simulink model "model2bf_Chikri"  (R2024b)
settings: Solver=ode4  StartTime=0.0  StopTime=20  FixedStep=2e-3  MaxStep=1e-1  RelTol=1e-3
values from neighbouring files (symbols this model uses):
  Aero = struct    [model2_dim.m]    (also in model2_dim_Chikri.m)
  brake = struct    [model2_dim.m]    (also in model2_dim_Chikri.m)
  drivetrain = struct    [model2_dim.m]    (also in model2_dim_Chikri.m)
  g = 9.81    [model2_dim.m]    (also in model2_dim_Chikri.m)
  G29 = struct    [model2_dim.m]    (also in model2_dim_Chikri.m)
  hub_offset = 2.5    [model2_dim.m]    (also in model2_dim_Chikri.m)
  motor = struct    [model2_dim.m]    (also in model2_dim_Chikri.m)
  slope_angle = 0    [model2_dim.m]    (also in model2_dim_Chikri.m)
  suspension = struct    [model2_dim.m]    (also in model2_dim_Chikri.m)
  tyre = struct    [model2_dim.m]    (also in model2_dim_Chikri.m)
  vehicle = struct    [Dimesnsion.m]    (also in model2_dim.m; model2_dim_Chikri.m)
undefined symbols (not defined in the file or in its folder): table, wheel, X, Y, Z
libraries: sm_lib x154, nesl_utility x46, simulink x8, slrealtimeG29lib x1, Contact_Forces_Lib x1
(part 1 of 6)
settings Model: Creator=francescovalentia  LastModifiedBy=chikr
settings SolverCC: ConcurrentTasks=on  SolverResetMethod=Robust  PositivePriorityOrder=on
settings DebuggingCC: ReadBeforeWriteMsg=DisableAll  WriteAfterWriteMsg=DisableAll  WriteAfterReadMsg=DisableAll  TasksWithSamePriorityMsg=none
settings HardwareCC: ProdBitPerLong=64  ProdLongLongMode=on  ProdHWDeviceType=Intel->x86-64 (Linux 64)
settings ModelReferenceCC: UpdateModelReferenceTargets=IfOutOfDate
settings SFSimCC: SFSimEcho=off
settings RTWCC: Description=Speedgoat Real-Time Target Machine  SystemTargetFile=speedgoat.tlc  TemplateMakefile=slrealtime_default_tmf  Toolchain=Simulink Real-Time Toolchain  BuildConfiguration=Faster Runs  CodeExecutionProfiling=on  TargetLang=C++
settings SimulinkRealTimeTargetCC: InstructionSetFMA=off  LogToMDFFile=off  SLRTForcePollingMode=on  UseGCCFastMath=on

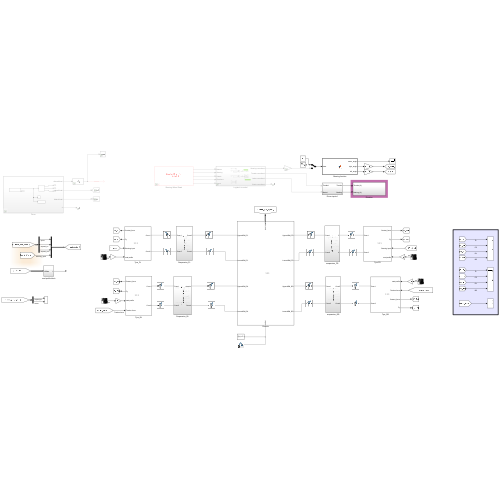
[thumbnail: Simulink's stored preview of the top-level diagram]
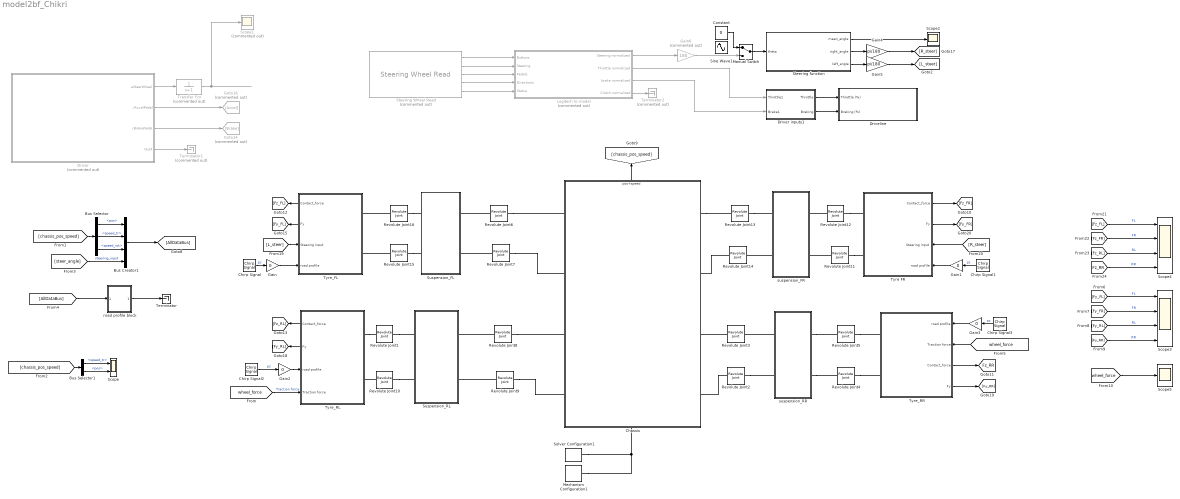
== system model2bf_Chikri ==
  Bus Creator1 : BusCreator  Inputs=4
  Bus Selector : BusSelector  OutputSignals=pos,speed_tr,speed_rot
  Bus Selector1 : BusSelector  OutputSignals=speed_tr,pos
  Chassis : Subsystem
      settings: PortSchema="{\"entries\":[{\"content\":{\"sides\":[{\"content\":{\"connectorIds\":[\"LConn1\",\"LConn2\",\"LConn3\",\"LConn4\"]},\"type\":\"ConnectorPlacement.EquallySpacedRectSide\",\"uuid\":\"90a4177c-ee01-4ca1-ac59-ac8cd2430efa\"},{\"content\":{\"connectorIds\":[\"RConn1\",\"RConn2\",\"RConn3\",\"RConn4\"],\"side\":\"RIGHT\"},\"type\":\"ConnectorPlacement.EquallySpacedRectSide\",\"uuid\":\"edda8be8-83bb-4564-b638-4691278f5470\"},{\"content\":{\"connectorIds\":[\"Out1\"],\"side\":\"TOP\"},\"type\":\"ConnectorPlacement.EquallySpacedRectSide\",\"uuid\":\"1072aa4a-3e89-42c9-923f-70cc607d97c1\"},{\"content\":{\"connectorIds\":[\"RConn5\"],\"side\":\"BOTTOM\"},\"type\":\"ConnectorPlacement.EquallySpacedRectSide\",\"uuid\":\"b3a5ffc1-0a8d-40b3-87bf-50b9fb640548\"}]},\"type\":\"ConnectorPlacement.EquallySpacedConnector\",\"uuid\":\"42fa0a11-996d-4d38-ac5b-1505bea5ca1e\"}],\"packageUris\":[\"http://schema.mathworks.com/mf0/Connector/R2020b\"],\"version\":\"1.0\"}"
      mask Display: image('Screenshot 2025-03-01 at 00.26 Background Removed.44.png');
  Chirp Signal{,1..3} (4 alike) : simulink/Sources/Chirp Signal  f1=0.01  T=10  f2=10
  Constant : Constant  Value=0
  Driveline : Subsystem
  Driver : Subsystem  Commented=on
  Driver inputs1 : Subsystem
  Gain{,1..3} (4 alike) : Gain  Gain=0
  Gain4 : Gain  Gain=pi/180
  Gain5 : Gain  Gain=pi/180
  Gain6 : Gain  Commented=on  Gain=180
  Goto14 : Goto  Commented=on  GotoTag=Brake
  Goto16 : Goto  Commented=on  GotoTag=Accel
  Logitech to model : Subsystem  Commented=on
  Manual Switch : ManualSwitch
  Mechanism Configuration1 : sm_lib/Utilities/Mechanism Configuration  UniformGravity=Constant  GravityVector=[0 0 -9.80665]  GravityVectorUnits=m/s^2  LinearizationDelta=0.001  JointModeTransitionNonlinearIterations=2
  Revolute Joint{1..16} (16 alike) : sm_lib/Joints/Revolute Joint  JointMode=Normal  CompositeWrenchDir=FollowerOnBase  CompositeWrenchFrame=BaseFrame  SenseConstraintForce=off  SenseConstraintTorque=off  SenseTotalForce=off  SenseTotalTorque=off  PositionTargetSpecify=off  PositionTargetPriority=High  PositionTargetValue=0  PositionTargetValueUnits=deg  VelocityTargetSpecify=off  VelocityTargetPriority=High  VelocityTargetValue=0  VelocityTargetValueUnits=deg/s  EquilibriumPosition=0  EquilibriumPositionUnits=deg  SpringStiffness=0  SpringStiffnessUnits=N*m/deg  DampingCoefficient=0  DampingCoefficientUnits=N*m/(deg/s)  LowerLimitSpecify=off  LowerLimitBound=-90  LowerLimitBoundUnits=deg  LowerLimitStiffness=1e4  LowerLimitStiffnessUnits=N*m/deg  LowerLimitDamping=10  LowerLimitDampingUnits=N*m/(deg/s)  LowerLimitTransitionRegionWidth=0.1  LowerLimitTransitionRegionWidthUnits=deg  UpperLimitSpecify=off  UpperLimitBound=90  UpperLimitBoundUnits=deg  UpperLimitStiffness=1e4  UpperLimitStiffnessUnits=N*m/deg  UpperLimitDamping=10  UpperLimitDampingUnits=N*m/(deg/s)  UpperLimitTransitionRegionWidth=0.1  UpperLimitTransitionRegionWidthUnits=deg  TorqueActuationMode=NoTorque  MotionActuationMode=ComputedMotion  SensePosition=off  SenseVelocity=off  SenseAcceleration=off  SenseTorqueForce=off  SenseLowerLimitTorqueForce=off  SenseUpperLimitTorqueForce=off
  Scope : Scope  NumInputPorts=2
  Scope1 : Scope  Commented=on
  Scope2 : Scope
  Scope3 : Scope  NumInputPorts=4
  Scope4 : Scope  NumInputPorts=4
  Scope5 : Scope
  Sine Wave1 : Sin  Amplitude=30  Frequency=1*2*pi  SampleTime=0
  Solver Configuration1 : nesl_utility/Solver Configuration  PhysicalDomain=network_engine_domain  SubClassName=solver  LeftPortType=input  RightPortType=generic  Tones=[]  Harmonics=[]  SimulateNoise=off  Profile=off  UseLocalSampling=off  EnableSwitchedLinearOptims=on  FrequencyDomain=off  UseCCode=off  RelTol=0.001  AbsTol=0.001  MinStep=1e-09  ToWorkspace=off  RevertToSquareIcSolve=off  NumHomotopyIterations=100  PhasorMode=off  PhasorModeNumHarmonics=1  ConsistencySolver=NEWTON_XTOL_AFTER_FTOL  IndexReductionMethod=DerivativeReplacement  DoDC=off  ResidualTolerance=1e-09  ConsistencyTolSource=GLOBAL  ConsistencyAbsTol=0.001  ConsistencyRelTol=0.001  ConsistencyTolFactor=0.02  UseLocalSolver=off  LocalSolverChoice=NE_BACKWARD_EULER_ADVANCER  ResolveIndetEquations=on  FunctionEvalNumThread=1  LocalSolverSampleTime=0.001  DoFixedCost=off  MaxNonlinIter=3  MaxModeIter=2  ComputeImpulses=off  ImpulseIterations=2  LinearAlgebra=auto  LinearAlgebraNumThread=0  EquationFormulation=NE_TIME_EF  DelaysMemoryBudget=1024  AutomaticFiltering=on  FilteringTimeConstant=0.001  PartitionStorageMethod=AS_NEEDED  PartitionMemoryBudget=1024  PartitionMethod=ROBUST  MultibodyUseLocalSolver=off  MultibodyLocalSolverChoice=ODE1  MultibodyLocalSolverSampleTime=0.001
  Steering Wheel Read : slrealtimeG29lib/Steering Wheel Read  Commented=on  sampleTime=-1
  Steering function : MATLAB Function  TreatAsAtomicUnit=on
  Suspension_FL : Subsystem
  Suspension_RL : Subsystem
  Terminator : Terminator
  Terminator1 : Terminator  Commented=on
  Terminator2 : Terminator  Commented=on
  Transfer Fcn : TransferFcn  Commented=on  Denominator=[1 1]
  Tyre FR : Subsystem
      settings: PortSchema="{\"entries\":[{\"content\":{\"sides\":[{\"content\":{\"connectorIds\":[\"LConn1\",\"LConn2\"]},\"type\":\"ConnectorPlacement.EquallySpacedRectSide\",\"uuid\":\"7590dd46-fd1e-41dd-87a1-62791c0994cf\"},{\"content\":{\"connectorIds\":[\"Out1\",\"Out2\",\"In1\",\"In2\"],\"side\":\"RIGHT\"},\"type\":\"ConnectorPlacement.EquallySpacedRectSide\",\"uuid\":\"4353fa18-87e5-46ea-8b75-e97175ca5d0d\"},{\"content\":{\"side\":\"TOP\"},\"type\":\"ConnectorPlacement.EquallySpacedRectSide\",\"uuid\":\"fb2fe8ac-4791-48d4-8005-7292892240b2\"}]},\"type\":\"ConnectorPlacement.EquallySpacedConnector\",\"uuid\":\"4af72fb6-bebe-4fb7-b2ff-d8311ffebfc8\"}],\"packageUris\":[\"http://schema.mathworks.com/mf0/Connector/R2020b\"],\"version\":\"1.0\"}"
      mask Display: image('tire.jpg');
  Tyre_FL : Subsystem
      settings: PortSchema="{\"entries\":[{\"content\":{\"sides\":[{\"content\":{\"connectorIds\":[\"Out1\",\"Out2\",\"In1\",\"In2\"]},\"type\":\"ConnectorPlacement.EquallySpacedRectSide\",\"uuid\":\"bd1bd92e-18de-4596-8220-631603715178\"},{\"content\":{\"connectorIds\":[\"RConn1\",\"RConn2\"],\"side\":\"RIGHT\"},\"type\":\"ConnectorPlacement.EquallySpacedRectSide\",\"uuid\":\"e020c9fe-d1b2-4d80-947d-230813d0e146\"},{\"content\":{\"side\":\"TOP\"},\"type\":\"ConnectorPlacement.EquallySpacedRectSide\",\"uuid\":\"ef1b0779-8900-451f-8b58-5aab45ce88d5\"}]},\"type\":\"ConnectorPlacement.EquallySpacedConnector\",\"uuid\":\"d082f1b5-3bbc-432b-b3b6-f4f290eb68cb\"}],\"packageUris\":[\"http://schema.mathworks.com/mf0/Connector/R2020b\"],\"version\":\"1.0\"}"
      mask Display: image('tire.jpg');
  Tyre_RL : Subsystem
      settings: PortSchema="{\"entries\":[{\"content\":{\"sides\":[{\"content\":{\"connectorIds\":[\"Out1\",\"Out2\",\"In1\",\"In2\"]},\"type\":\"ConnectorPlacement.EquallySpacedRectSide\",\"uuid\":\"bd1bd92e-18de-4596-8220-631603715178\"},{\"content\":{\"connectorIds\":[\"RConn1\",\"RConn2\"],\"side\":\"RIGHT\"},\"type\":\"ConnectorPlacement.EquallySpacedRectSide\",\"uuid\":\"e020c9fe-d1b2-4d80-947d-230813d0e146\"},{\"content\":{\"side\":\"TOP\"},\"type\":\"ConnectorPlacement.EquallySpacedRectSide\",\"uuid\":\"ef1b0779-8900-451f-8b58-5aab45ce88d5\"}]},\"type\":\"ConnectorPlacement.EquallySpacedConnector\",\"uuid\":\"d082f1b5-3bbc-432b-b3b6-f4f290eb68cb\"}],\"packageUris\":[\"http://schema.mathworks.com/mf0/Connector/R2020b\"],\"version\":\"1.0\"}"
      mask Display: image('tire.jpg');
  Tyre_RR : Subsystem
      settings: PortSchema="{\"entries\":[{\"content\":{\"sides\":[{\"content\":{\"connectorIds\":[\"LConn1\",\"LConn2\"]},\"type\":\"ConnectorPlacement.EquallySpacedRectSide\",\"uuid\":\"a564fd7b-0f32-4e80-8b02-b8b45a5adc28\"},{\"content\":{\"connectorIds\":[\"In1\",\"In2\",\"Out1\",\"Out2\"],\"side\":\"RIGHT\"},\"type\":\"ConnectorPlacement.EquallySpacedRectSide\",\"uuid\":\"62803d7e-dbc7-484c-b5fe-641aa1e4ceba\"},{\"content\":{\"side\":\"TOP\"},\"type\":\"ConnectorPlacement.EquallySpacedRectSide\",\"uuid\":\"ba4bb9da-1b26-49aa-a650-9164e637a846\"}]},\"type\":\"ConnectorPlacement.EquallySpacedConnector\",\"uuid\":\"c0290aae-2bf5-4993-a041-c2ed20fa197e\"}],\"packageUris\":[\"http://schema.mathworks.com/mf0/Connector/R2020b\"],\"version\":\"1.0\"}"
      mask Display: image('tire.jpg');
  road profile block : Subsystem
  suspension_FR : Subsystem
  suspension_RR : Subsystem
  tag scope: Fz_RR=global
  wires:
  Chirp Signal/1 -> Gain/1  "pz"
  Gain/1 -> Tyre_FL/2(road profile)
  Bus Creator1/1 -> [AllDataBus]
  [AllDataBus] -> road profile block/1(Alldata)
  road profile block/1(Out1) -> Terminator/1
  Gain1/1 -> Tyre FR/2(road profile)
  Chirp Signal1/1 -> Gain1/1  "pz"
  Chirp Signal2/1 -> Gain2/1  "pz"
  Gain2/1 -> Tyre_RL/1(road profile)
  Chirp Signal3/1 -> Gain3/1  "pz"
  Gain3/1 -> Tyre_RR/1(road profile)
  Chassis/1(pos+speed) -> [chassis_pos_speed]
  [steer_angle] -> Bus Creator1/4  "steering_input"
  [chassis_pos_speed] -> Bus Selector/1
  Bus Selector/1 -> Bus Creator1/1  "<pos>"
  [chassis_pos_speed] -> Bus Selector1/1
  Bus Selector1/1 -> Scope/1  "<speed_tr>"
  Tyre FR/1(Contact_force) -> [Fz_FR]
  Tyre_RR/1(Contact_force) -> [Fz_RR]
  Tyre_FL/1(Contact_force) -> [Fz_FL]
  Tyre_RL/1(Contact_force) -> [Fz_RL]
  [L_steer] -> Tyre_FL/1(Steering input)
  [R_steer] -> Tyre FR/1(Steering input)
  Transfer Fcn/1 -> Scope1/1
  Driver/2(rAccelPedal) -> Goto16/1
  Driver/1(aSteerWheel) -> Transfer Fcn/1
  Driver/4(Out4) -> Terminator1/1
  Driver/3(rBrakePedal) -> Goto14/1
  [Fz_FL] -> Scope4/1  "FL"
  [Fz_FR] -> Scope4/2  "FR"
  [Fz_RL] -> Scope4/3  "RL"
  [Fz_RR] -> Scope4/4  "RR"
  Steering function/3(left_angle) -> Gain5/1
  Steering function/2(right_angle) -> Gain4/1
  Bus Selector1/2 -> Scope/2  "<pos>"
  Bus Selector/2 -> Bus Creator1/2  "<speed_tr>"
  Bus Selector/3 -> Bus Creator1/3  "<speed_rot>"
  [wheel_force] -> Tyre_RL/2(Traction force)  "Traction force"
  [wheel_force] -> Tyre_RR/2(Traction force)
  Steering function/1(mean_angle) -> Scope2/1
  Gain4/1 -> [R_steer]
  Gain5/1 -> [L_steer]
  [Fy_FR] -> Scope3/2  "FR"
  [Fy_RL] -> Scope3/3  "RL"
  [Fy_FL] -> Scope3/1  "FL"
  [Fy_RR] -> Scope3/4  "RR"
  Tyre_FL/2(Fy) -> [Fy_FL]
  Tyre_RL/2(Fy) -> [Fy_RL]
  Tyre_RR/2(Fy) -> [Fy_RR]
  Tyre FR/2(Fy) -> [Fy_FR]
  [wheel_force] -> Scope5/1
  Steering Wheel Read/1 -> Logitech to model/1(Buttons)
  Steering Wheel Read/2 -> Logitech to model/2(Steering)
  Steering Wheel Read/3 -> Logitech to model/3(Pedals)
  Steering Wheel Read/4 -> Logitech to model/4(Directions)
  Steering Wheel Read/5 -> Logitech to model/5(Status)
  Logitech to model/1(Steering normalized) -> Gain6/1
  Logitech to model/4(Clutch normalized) -> Terminator2/1
  Driver inputs1/1(Throttle) -> Driveline/1(Throttle (%))
  Driver inputs1/2(Braking) -> Driveline/2(Braking (%))
  Manual Switch/1 -> Steering function/1(theta)
  Gain6/1 -> Manual Switch/2
  Logitech to model/2(Throttle normalized) -> Driver inputs1/1(Throttle1)
  Logitech to model/3(brake normalized) -> Driver inputs1/2(Brake1)
  Constant/1 -> Manual Switch/1
  connections:
  Solver Configuration1/RConn1 -- Mechanism Configuration1/RConn1 -- Chassis/RConn5
  Revolute Joint3/LConn1 -- Chassis/RConn3
  Revolute Joint2/LConn1 -- Chassis/RConn4
  Revolute Joint7/RConn1 -- Chassis/LConn2
  suspension_RR/LConn1 -- Revolute Joint3/RConn1
  Revolute Joint2/RConn1 -- suspension_RR/LConn2
  suspension_RR/RConn2 -- Revolute Joint4/LConn1
  suspension_RR/RConn1 -- Revolute Joint5/LConn1
  Revolute Joint12/LConn1 -- suspension_FR/RConn1
  Revolute Joint11/LConn1 -- suspension_FR/RConn2
  Revolute Joint14/LConn1 -- Chassis/RConn2
  suspension_FR/LConn2 -- Revolute Joint14/RConn1
  Chassis/RConn1 -- Revolute Joint13/LConn1
  Revolute Joint13/RConn1 -- suspension_FR/LConn1
  Revolute Joint12/RConn1 -- Tyre FR/LConn1
  Revolute Joint11/RConn1 -- Tyre FR/LConn2
  Revolute Joint16/RConn1 -- Tyre_FL/RConn1
  Revolute Joint15/RConn1 -- Tyre_FL/RConn2
  Tyre_RL/RConn1 -- Revolute Joint1/LConn1
  Revolute Joint10/LConn1 -- Tyre_RL/RConn2
  Revolute Joint1/RConn1 -- Suspension_RL/LConn1
  Revolute Joint8/LConn1 -- Suspension_RL/RConn1
  Revolute Joint10/RConn1 -- Suspension_RL/LConn2
  Revolute Joint9/LConn1 -- Suspension_RL/RConn2
  Revolute Joint16/LConn1 -- Suspension_FL/LConn1
  Revolute Joint6/LConn1 -- Suspension_FL/RConn1
  Revolute Joint15/LConn1 -- Suspension_FL/LConn2
  Revolute Joint7/LConn1 -- Suspension_FL/RConn2
  Revolute Joint8/RConn1 -- Chassis/LConn3
  Revolute Joint9/RConn1 -- Chassis/LConn4
  Revolute Joint6/RConn1 -- Chassis/LConn1
  Revolute Joint5/RConn1 -- Tyre_RR/LConn1
  Revolute Joint4/RConn1 -- Tyre_RR/LConn2

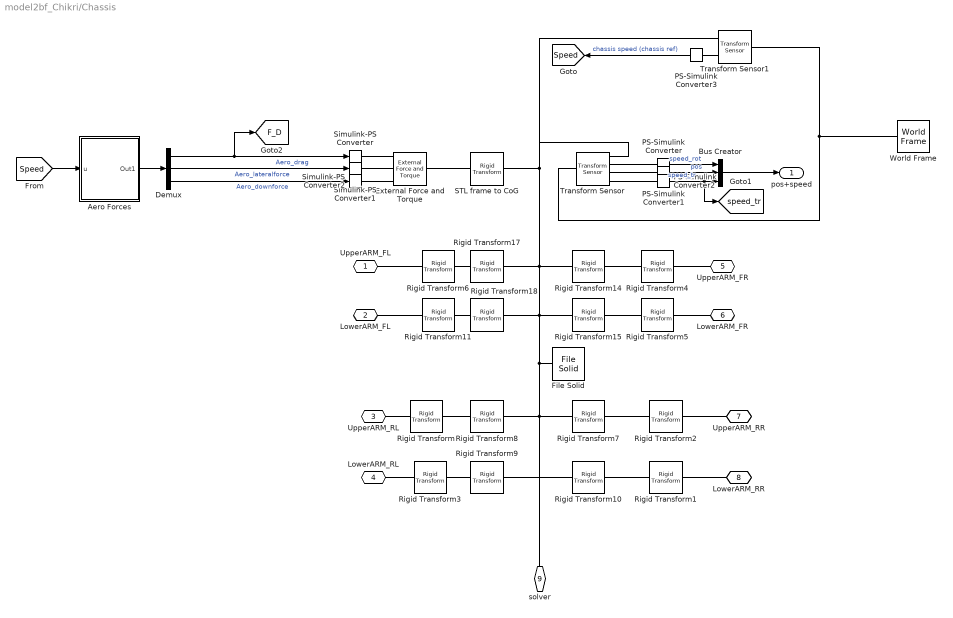
== system model2bf_Chikri/Chassis ==
  Aero Forces : Subsystem
  Bus Creator : BusCreator  Inputs=3
  Demux : Demux  Outputs=3
  External Force and Torque : sm_lib/Forces and Torques/External Force and Torque  EnableForceX=on  EnableForceY=on  EnableForceZ=on  EnableForce=off  ForceResolutionFrame=AttachedFrame  EnableTorqueX=off  EnableTorqueY=off  EnableTorqueZ=off  EnableTorque=off  TorqueResolutionFrame=AttachedFrame
  File Solid : sm_lib/Body Elements/File Solid  ExtGeomFileName=C:\Users\chikr\Documents\formula\FRAME_KMLI.STL  UnitType=Custom  ExtGeomFileUnits=mm  StepReaderType=HEX  ExportConvexHullGeometry=off  InertiaType=CalculateFromGeometry  BasedOnType=Density  Density=7850  DensityUnits=kg/m^3  Mass=1  MassUnits=kg  CenterOfMass=[0 0 0]  CenterOfMassUnits=m  MomentsOfInertia=[1 1 1]  MomentsOfInertiaUnits=kg*m^2  ProductsOfInertia=[0 0 0]  ProductsOfInertiaUnits=kg*m^2  GraphicType=FromGeometry  MarkerShape=Sphere  MarkerSize=10  GraphicVisPropType=SimpleVisualProperties  GraphicDiffuseColor=[0.5 0.5 0.5]  GraphicOpacity=1  GraphicSpecularColor=[0.5 0.5 0.5 1.0]  GraphicAmbientColor=[0.15 0.15 0.15 1.0]  GraphicEmissiveColor=[0.0 0.0 0.0 1.0]  GraphicShininess=75  DoExposeReferenceFrame=on  SerializedFrames=<Frames/>
  PS-Simulink Converter{,1..3} (4 alike) : nesl_utility/PS-Simulink Converter  PhysicalDomain=network_engine_domain  SubClassName=ps_output  LeftPortType=input  RightPortType=output  PseudoPeriodic=off  Frequencies=[]  VectorFormat=inherit  Unit=inherit  AffineConversion=off
  Rigid Transform : sm_lib/Frames and Transforms/Rigid Transform  RotationMethod=StandardAxis  FollAlignAxisA=+X  BaseAlignAxisA=+Y  FollAlignAxisB=+Y  BaseAlignAxisB=+Z  RotationStandardAxis=-Z  RotationAngle=suspension.rear.upper.inclination  RotationAngleUnits=deg  RotationArbitraryAxis=[0 0 1]  RotationSequenceAxes=FollowerAxes  RotationSequence=XYX  RotationSequenceAngles=[0 0 0]  RotationSequenceAnglesUnits=deg  RotationMatrix=[1 0 0;0 1 0;0 0 1]  Quaternion=[1 0 0 0]  TranslationMethod=None  TranslationCartesianOffset=[0 0 0]  TranslationCartesianOffsetUnits=m  TranslationStandardAxis=+Z  TranslationStandardOffset=0  TranslationStandardOffsetUnits=m  TranslationROffset=0  TranslationROffsetUnits=m  TranslationThetaOffset=0  TranslationThetaOffsetUnits=deg  TranslationZOffset=0  TranslationZOffsetUnits=m
  Rigid Transform1 : sm_lib/Frames and Transforms/Rigid Transform  RotationMethod=StandardAxis  FollAlignAxisA=+X  BaseAlignAxisA=+Y  FollAlignAxisB=+Y  BaseAlignAxisB=+Z  RotationStandardAxis=+Z  RotationAngle=suspension.rear.lower.inclination  RotationAngleUnits=deg  RotationArbitraryAxis=[0 0 1]  RotationSequenceAxes=FollowerAxes  RotationSequence=XYX  RotationSequenceAngles=[0 0 0]  RotationSequenceAnglesUnits=deg  RotationMatrix=[1 0 0;0 1 0;0 0 1]  Quaternion=[1 0 0 0]  TranslationMethod=None  TranslationCartesianOffset=[0 -suspension.rear.lower.length/2 0]  TranslationCartesianOffsetUnits=cm  TranslationStandardAxis=+Z  TranslationStandardOffset=0  TranslationStandardOffsetUnits=m  TranslationROffset=0  TranslationROffsetUnits=m  TranslationThetaOffset=0  TranslationThetaOffsetUnits=deg  TranslationZOffset=0  TranslationZOffsetUnits=m
  Rigid Transform10 : sm_lib/Frames and Transforms/Rigid Transform  RotationMethod=StandardAxis  FollAlignAxisA=+X  BaseAlignAxisA=+Y  FollAlignAxisB=+Y  BaseAlignAxisB=+Z  RotationStandardAxis=+Y  RotationAngle=90  RotationAngleUnits=deg  RotationArbitraryAxis=[0 0 1]  RotationSequenceAxes=FollowerAxes  RotationSequence=XYX  RotationSequenceAngles=[0 0 0]  RotationSequenceAnglesUnits=deg  RotationMatrix=[1 0 0;0 1 0;0 0 1]  Quaternion=[1 0 0 0]  TranslationMethod=Cartesian  TranslationCartesianOffset=[173 -160 0]  TranslationCartesianOffsetUnits=mm  TranslationStandardAxis=+Z  TranslationStandardOffset=0  TranslationStandardOffsetUnits=m  TranslationROffset=0  TranslationROffsetUnits=m  TranslationThetaOffset=0  TranslationThetaOffsetUnits=deg  TranslationZOffset=0  TranslationZOffsetUnits=m
  Rigid Transform11 : sm_lib/Frames and Transforms/Rigid Transform  RotationMethod=StandardAxis  FollAlignAxisA=+X  BaseAlignAxisA=+Y  FollAlignAxisB=+Y  BaseAlignAxisB=+Z  RotationStandardAxis=-Z  RotationAngle=suspension.front.lower.inclination  RotationAngleUnits=deg  RotationArbitraryAxis=[0 0 1]  RotationSequenceAxes=FollowerAxes  RotationSequence=XYX  RotationSequenceAngles=[0 0 0]  RotationSequenceAnglesUnits=deg  RotationMatrix=[1 0 0;0 1 0;0 0 1]  Quaternion=[1 0 0 0]  TranslationMethod=None  TranslationCartesianOffset=[0 -suspension.rear.lower.length/2 0]  TranslationCartesianOffsetUnits=cm  TranslationStandardAxis=+Z  TranslationStandardOffset=0  TranslationStandardOffsetUnits=m  TranslationROffset=0  TranslationROffsetUnits=m  TranslationThetaOffset=0  TranslationThetaOffsetUnits=deg  TranslationZOffset=0  TranslationZOffsetUnits=m
  Rigid Transform14 : sm_lib/Frames and Transforms/Rigid Transform  RotationMethod=StandardAxis  FollAlignAxisA=+X  BaseAlignAxisA=+Y  FollAlignAxisB=+Y  BaseAlignAxisB=+Z  RotationStandardAxis=+Y  RotationAngle=90  RotationAngleUnits=deg  RotationArbitraryAxis=[0 0 1]  RotationSequenceAxes=FollowerAxes  RotationSequence=XYX  RotationSequenceAngles=[0 0 0]  RotationSequenceAnglesUnits=deg  RotationMatrix=[1 0 0;0 1 0;0 0 1]  Quaternion=[1 0 0 0]  TranslationMethod=Cartesian  TranslationCartesianOffset=[1720 -232 202]  TranslationCartesianOffsetUnits=mm  TranslationStandardAxis=+Z  TranslationStandardOffset=0  TranslationStandardOffsetUnits=m  TranslationROffset=0  TranslationROffsetUnits=m  TranslationThetaOffset=0  TranslationThetaOffsetUnits=deg  TranslationZOffset=0  TranslationZOffsetUnits=m
  Rigid Transform15 : sm_lib/Frames and Transforms/Rigid Transform  RotationMethod=StandardAxis  FollAlignAxisA=+X  BaseAlignAxisA=+Y  FollAlignAxisB=+Y  BaseAlignAxisB=+Z  RotationStandardAxis=+Y  RotationAngle=90  RotationAngleUnits=deg  RotationArbitraryAxis=[0 0 1]  RotationSequenceAxes=FollowerAxes  RotationSequence=XYX  RotationSequenceAngles=[0 0 0]  RotationSequenceAnglesUnits=deg  RotationMatrix=[1 0 0;0 1 0;0 0 1]  Quaternion=[1 0 0 0]  TranslationMethod=Cartesian  TranslationCartesianOffset=[1720 -244 0]  TranslationCartesianOffsetUnits=mm  TranslationStandardAxis=+Z  TranslationStandardOffset=0  TranslationStandardOffsetUnits=m  TranslationROffset=0  TranslationROffsetUnits=m  TranslationThetaOffset=0  TranslationThetaOffsetUnits=deg  TranslationZOffset=0  TranslationZOffsetUnits=m
  Rigid Transform17 : sm_lib/Frames and Transforms/Rigid Transform  RotationMethod=StandardAxis  FollAlignAxisA=+X  BaseAlignAxisA=+Y  FollAlignAxisB=+Y  BaseAlignAxisB=+Z  RotationStandardAxis=+Y  RotationAngle=90  RotationAngleUnits=deg  RotationArbitraryAxis=[0 0 1]  RotationSequenceAxes=FollowerAxes  RotationSequence=XYX  RotationSequenceAngles=[0 0 0]  RotationSequenceAnglesUnits=deg  RotationMatrix=[1 0 0;0 1 0;0 0 1]  Quaternion=[1 0 0 0]  TranslationMethod=Cartesian  TranslationCartesianOffset=[1720 232 202]  TranslationCartesianOffsetUnits=mm  TranslationStandardAxis=+Z  TranslationStandardOffset=0  TranslationStandardOffsetUnits=m  TranslationROffset=0  TranslationROffsetUnits=m  TranslationThetaOffset=0  TranslationThetaOffsetUnits=deg  TranslationZOffset=0  TranslationZOffsetUnits=m
  Rigid Transform18 : sm_lib/Frames and Transforms/Rigid Transform  RotationMethod=StandardAxis  FollAlignAxisA=+X  BaseAlignAxisA=+Y  FollAlignAxisB=+Y  BaseAlignAxisB=+Z  RotationStandardAxis=+Y  RotationAngle=90  RotationAngleUnits=deg  RotationArbitraryAxis=[0 0 1]  RotationSequenceAxes=FollowerAxes  RotationSequence=XYX  RotationSequenceAngles=[0 0 0]  RotationSequenceAnglesUnits=deg  RotationMatrix=[1 0 0;0 1 0;0 0 1]  Quaternion=[1 0 0 0]  TranslationMethod=Cartesian  TranslationCartesianOffset=[1720 244 0]  TranslationCartesianOffsetUnits=mm  TranslationStandardAxis=+Z  TranslationStandardOffset=0  TranslationStandardOffsetUnits=m  TranslationROffset=0  TranslationROffsetUnits=m  TranslationThetaOffset=0  TranslationThetaOffsetUnits=deg  TranslationZOffset=0  TranslationZOffsetUnits=m
  Rigid Transform2 : sm_lib/Frames and Transforms/Rigid Transform  RotationMethod=StandardAxis  FollAlignAxisA=+X  BaseAlignAxisA=+Y  FollAlignAxisB=+Y  BaseAlignAxisB=+Z  RotationStandardAxis=+Z  RotationAngle=suspension.rear.upper.inclination  RotationAngleUnits=deg  RotationArbitraryAxis=[0 0 1]  RotationSequenceAxes=FollowerAxes  RotationSequence=XYX  RotationSequenceAngles=[0 0 0]  RotationSequenceAnglesUnits=deg  RotationMatrix=[1 0 0;0 1 0;0 0 1]  Quaternion=[1 0 0 0]  TranslationMethod=None  TranslationCartesianOffset=[0 -suspension.rear.lower.length/2 0]  TranslationCartesianOffsetUnits=cm  TranslationStandardAxis=+Z  TranslationStandardOffset=0  TranslationStandardOffsetUnits=m  TranslationROffset=0  TranslationROffsetUnits=m  TranslationThetaOffset=0  TranslationThetaOffsetUnits=deg  TranslationZOffset=0  TranslationZOffsetUnits=m
  Rigid Transform3 : sm_lib/Frames and Transforms/Rigid Transform  RotationMethod=StandardAxis  FollAlignAxisA=+X  BaseAlignAxisA=+Y  FollAlignAxisB=+Y  BaseAlignAxisB=+Z  RotationStandardAxis=-Z  RotationAngle=suspension.rear.lower.inclination  RotationAngleUnits=deg  RotationArbitraryAxis=[0 0 1]  RotationSequenceAxes=FollowerAxes  RotationSequence=XYX  RotationSequenceAngles=[0 0 0]  RotationSequenceAnglesUnits=deg  RotationMatrix=[1 0 0;0 1 0;0 0 1]  Quaternion=[1 0 0 0]  TranslationMethod=None  TranslationCartesianOffset=[0 0 0]  TranslationCartesianOffsetUnits=m  TranslationStandardAxis=+Z  TranslationStandardOffset=0  TranslationStandardOffsetUnits=m  TranslationROffset=0  TranslationROffsetUnits=m  TranslationThetaOffset=0  TranslationThetaOffsetUnits=deg  TranslationZOffset=0  TranslationZOffsetUnits=m
  Rigid Transform4 : sm_lib/Frames and Transforms/Rigid Transform  RotationMethod=StandardAxis  FollAlignAxisA=+X  BaseAlignAxisA=+Y  FollAlignAxisB=+Y  BaseAlignAxisB=+Z  RotationStandardAxis=+Z  RotationAngle=suspension.front.upper.inclination  RotationAngleUnits=deg  RotationArbitraryAxis=[0 0 1]  RotationSequenceAxes=FollowerAxes  RotationSequence=XYX  RotationSequenceAngles=[0 0 0]  RotationSequenceAnglesUnits=deg  RotationMatrix=[1 0 0;0 1 0;0 0 1]  Quaternion=[1 0 0 0]  TranslationMethod=None  TranslationCartesianOffset=[0 -suspension.rear.lower.length/2 0]  TranslationCartesianOffsetUnits=cm  TranslationStandardAxis=+Z  TranslationStandardOffset=0  TranslationStandardOffsetUnits=m  TranslationROffset=0  TranslationROffsetUnits=m  TranslationThetaOffset=0  TranslationThetaOffsetUnits=deg  TranslationZOffset=0  TranslationZOffsetUnits=m
  Rigid Transform5 : sm_lib/Frames and Transforms/Rigid Transform  RotationMethod=StandardAxis  FollAlignAxisA=+X  BaseAlignAxisA=+Y  FollAlignAxisB=+Y  BaseAlignAxisB=+Z  RotationStandardAxis=+Z  RotationAngle=suspension.front.lower.inclination  RotationAngleUnits=deg  RotationArbitraryAxis=[0 0 1]  RotationSequenceAxes=FollowerAxes  RotationSequence=XYX  RotationSequenceAngles=[0 0 0]  RotationSequenceAnglesUnits=deg  RotationMatrix=[1 0 0;0 1 0;0 0 1]  Quaternion=[1 0 0 0]  TranslationMethod=None  TranslationCartesianOffset=[0 -suspension.rear.lower.length/2 0]  TranslationCartesianOffsetUnits=cm  TranslationStandardAxis=+Z  TranslationStandardOffset=0  TranslationStandardOffsetUnits=m  TranslationROffset=0  TranslationROffsetUnits=m  TranslationThetaOffset=0  TranslationThetaOffsetUnits=deg  TranslationZOffset=0  TranslationZOffsetUnits=m
  Rigid Transform6 : sm_lib/Frames and Transforms/Rigid Transform  RotationMethod=StandardAxis  FollAlignAxisA=+X  BaseAlignAxisA=+Y  FollAlignAxisB=+Y  BaseAlignAxisB=+Z  RotationStandardAxis=+Z  RotationAngle=suspension.rear.lower.inclination  RotationAngleUnits=deg  RotationArbitraryAxis=[0 0 1]  RotationSequenceAxes=FollowerAxes  RotationSequence=XYX  RotationSequenceAngles=[0 0 0]  RotationSequenceAnglesUnits=deg  RotationMatrix=[1 0 0;0 1 0;0 0 1]  Quaternion=[1 0 0 0]  TranslationMethod=None  TranslationCartesianOffset=[0 -suspension.rear.lower.length/2 0]  TranslationCartesianOffsetUnits=cm  TranslationStandardAxis=+Z  TranslationStandardOffset=0  TranslationStandardOffsetUnits=m  TranslationROffset=0  TranslationROffsetUnits=m  TranslationThetaOffset=0  TranslationThetaOffsetUnits=deg  TranslationZOffset=0  TranslationZOffsetUnits=m
  Rigid Transform7 : sm_lib/Frames and Transforms/Rigid Transform  RotationMethod=StandardAxis  FollAlignAxisA=+X  BaseAlignAxisA=+Y  FollAlignAxisB=+Y  BaseAlignAxisB=+Z  RotationStandardAxis=+Y  RotationAngle=90  RotationAngleUnits=deg  RotationArbitraryAxis=[0 0 1]  RotationSequenceAxes=FollowerAxes  RotationSequence=XYX  RotationSequenceAngles=[0 0 0]  RotationSequenceAnglesUnits=deg  RotationMatrix=[1 0 0;0 1 0;0 0 1]  Quaternion=[1 0 0 0]  TranslationMethod=Cartesian  TranslationCartesianOffset=[173 -160 205]  TranslationCartesianOffsetUnits=mm  TranslationStandardAxis=+Z  TranslationStandardOffset=0  TranslationStandardOffsetUnits=m  TranslationROffset=0  TranslationROffsetUnits=m  TranslationThetaOffset=0  TranslationThetaOffsetUnits=deg  TranslationZOffset=0  TranslationZOffsetUnits=m
  Rigid Transform8 : sm_lib/Frames and Transforms/Rigid Transform  RotationMethod=StandardAxis  FollAlignAxisA=+X  BaseAlignAxisA=+Y  FollAlignAxisB=+Y  BaseAlignAxisB=+Z  RotationStandardAxis=+Y  RotationAngle=90  RotationAngleUnits=deg  RotationArbitraryAxis=[0 0 1]  RotationSequenceAxes=FollowerAxes  RotationSequence=XYX  RotationSequenceAngles=[0 0 0]  RotationSequenceAnglesUnits=deg  RotationMatrix=[1 0 0;0 1 0;0 0 1]  Quaternion=[1 0 0 0]  TranslationMethod=Cartesian  TranslationCartesianOffset=[173 160 205]  TranslationCartesianOffsetUnits=mm  TranslationStandardAxis=+Z  TranslationStandardOffset=0  TranslationStandardOffsetUnits=m  TranslationROffset=0  TranslationROffsetUnits=m  TranslationThetaOffset=0  TranslationThetaOffsetUnits=deg  TranslationZOffset=0  TranslationZOffsetUnits=m
  Rigid Transform9 : sm_lib/Frames and Transforms/Rigid Transform  RotationMethod=StandardAxis  FollAlignAxisA=+X  BaseAlignAxisA=+Y  FollAlignAxisB=+Y  BaseAlignAxisB=+Z  RotationStandardAxis=+Y  RotationAngle=90  RotationAngleUnits=deg  RotationArbitraryAxis=[0 0 1]  RotationSequenceAxes=FollowerAxes  RotationSequence=XYX  RotationSequenceAngles=[0 0 0]  RotationSequenceAnglesUnits=deg  RotationMatrix=[1 0 0;0 1 0;0 0 1]  Quaternion=[1 0 0 0]  TranslationMethod=Cartesian  TranslationCartesianOffset=[173 160 0]  TranslationCartesianOffsetUnits=mm  TranslationStandardAxis=+Z  TranslationStandardOffset=0  TranslationStandardOffsetUnits=m  TranslationROffset=0  TranslationROffsetUnits=m  TranslationThetaOffset=0  TranslationThetaOffsetUnits=deg  TranslationZOffset=0  TranslationZOffsetUnits=m
  STL frame to CoG : sm_lib/Frames and Transforms/Rigid Transform  RotationMethod=None  FollAlignAxisA=+X  BaseAlignAxisA=+Y  FollAlignAxisB=+Y  BaseAlignAxisB=+Z  RotationStandardAxis=+Z  RotationAngle=0  RotationAngleUnits=deg  RotationArbitraryAxis=[0 0 1]  RotationSequenceAxes=FollowerAxes  RotationSequence=XYX  RotationSequenceAngles=[0 0 0]  RotationSequenceAnglesUnits=deg  RotationMatrix=[1 0 0;0 1 0;0 0 1]  Quaternion=[1 0 0 0]  TranslationMethod=Cartesian  TranslationCartesianOffset=[0.966323 -0.000859 0.18232]  TranslationCartesianOffsetUnits=m  TranslationStandardAxis=+Z  TranslationStandardOffset=0  TranslationStandardOffsetUnits=m  TranslationROffset=0  TranslationROffsetUnits=m  TranslationThetaOffset=0  TranslationThetaOffsetUnits=deg  TranslationZOffset=0  TranslationZOffsetUnits=m
  Simulink-PS Converter : nesl_utility/Simulink-PS Converter  PhysicalDomain=network_engine_domain  SubClassName=ps_input  LeftPortType=input  RightPortType=output  PseudoPeriodic=off  Frequencies=[]  NoiseDistribution=none  NoiseParameters=[]  Unit=1  AffineConversion=off  FilteringAndDerivatives=provide  SimscapeFilterOrder=1  InputFilterTimeConstant=0.001  UdotUserProvided=0
  Simulink-PS Converter1 : nesl_utility/Simulink-PS Converter  PhysicalDomain=network_engine_domain  SubClassName=ps_input  LeftPortType=input  RightPortType=output  PseudoPeriodic=off  Frequencies=[]  NoiseDistribution=none  NoiseParameters=[]  Unit=1  AffineConversion=off  FilteringAndDerivatives=provide  SimscapeFilterOrder=1  InputFilterTimeConstant=0.001  UdotUserProvided=0
  Simulink-PS Converter2 : nesl_utility/Simulink-PS Converter  PhysicalDomain=network_engine_domain  SubClassName=ps_input  LeftPortType=input  RightPortType=output  PseudoPeriodic=off  Frequencies=[]  NoiseDistribution=none  NoiseParameters=[]  Unit=1  AffineConversion=off  FilteringAndDerivatives=provide  SimscapeFilterOrder=1  InputFilterTimeConstant=0.001  UdotUserProvided=0
  Transform Sensor : sm_lib/Frames and Transforms/Transform Sensor  MeasurementFrame=World  RotationSequence=XYZ  SenseAngle=off  SenseAxis=off  SenseQ=off  SenseR=off  SenseRotationSequence=off  SenseOmegaX=off  SenseOmegaY=off  SenseOmegaZ=off  SenseOmega=on  SenseQDot=off  SenseRDot=off  SenseRotationSequenceDot=off  SenseAlphaX=off  SenseAlphaY=off  SenseAlphaZ=off  SenseAlpha=off  SenseQDDot=off  SenseRDDot=off  SenseX=off  SenseY=off  SenseZ=off  SenseXYZ=on  SenseRad=off  SenseAzim=off  SenseDist=off  SenseInc=off  SenseXDot=off  SenseYDot=off  SenseZDot=off  SenseXYZDot=on  SenseRadDot=off  SenseAzimDot=off  SenseDistDot=off  SenseIncDot=off  SenseXDDot=off  SenseYDDot=off  SenseZDDot=off  SenseXYZDDot=off  SenseRadDDot=off  SenseAzimDDot=off  SenseDistDDot=off  SenseIncDDot=off
  Transform Sensor1 : sm_lib/Frames and Transforms/Transform Sensor  MeasurementFrame=Follower  RotationSequence=XYZ  SenseAngle=off  SenseAxis=off  SenseQ=off  SenseR=off  SenseRotationSequence=off  SenseOmegaX=off  SenseOmegaY=off  SenseOmegaZ=off  SenseOmega=off  SenseQDot=off  SenseRDot=off  SenseRotationSequenceDot=off  SenseAlphaX=off  SenseAlphaY=off  SenseAlphaZ=off  SenseAlpha=off  SenseQDDot=off  SenseRDDot=off  SenseX=off  SenseY=off  SenseZ=off  SenseXYZ=off  SenseRad=off  SenseAzim=off  SenseDist=off  SenseInc=off  SenseXDot=off  SenseYDot=off  SenseZDot=off  SenseXYZDot=on  SenseRadDot=off  SenseAzimDot=off  SenseDistDot=off  SenseIncDot=off  SenseXDDot=off  SenseYDDot=off  SenseZDDot=off  SenseXYZDDot=off  SenseRadDDot=off  SenseAzimDDot=off  SenseDistDDot=off  SenseIncDDot=off
  World Frame : sm_lib/Frames and Transforms/World Frame
  UpperARM_FL : PMIOPort  Side=Left
  LowerARM_FL : PMIOPort  Port=2  Side=Left
  UpperARM_RL : PMIOPort  Port=3  Side=Left
  LowerARM_RL : PMIOPort  Port=4  Side=Left
  UpperARM_FR : PMIOPort  Port=5  Side=Right
  LowerARM_FR : PMIOPort  Port=6  Side=Right
  UpperARM_RR : PMIOPort  Port=7  Side=Right
  LowerARM_RR : PMIOPort  Port=8  Side=Right
  solver : PMIOPort  Port=9  Side=Right
  pos+speed : Outport
  tag scope: F_D=global, Speed=global, speed_tr=global
  wires:
  Demux/1 -> [F_D], Simulink-PS Converter/1  "Aero_drag"
  Demux/2 -> Simulink-PS Converter1/1  "Aero_lateralforce"
  Demux/3 -> Simulink-PS Converter2/1  "Aero_downforce"
  PS-Simulink Converter/1 -> Bus Creator/1  "speed_rot"
  PS-Simulink Converter1/1 -> Bus Creator/2  "pos"
  Bus Creator/1 -> pos+speed/1
  PS-Simulink Converter2/1 -> [speed_tr], Bus Creator/3  "speed_tr"
  [Speed] -> Aero Forces/1(u)
  Aero Forces/1(Out1) -> Demux/1
  PS-Simulink Converter3/1 -> [Speed]  "chassis speed (chassis ref)"
  connections:
  Rigid Transform/RConn1 -- UpperARM_RL/RConn1
  UpperARM_RR/RConn1 -- Rigid Transform2/RConn1
  Rigid Transform3/RConn1 -- LowerARM_RL/RConn1
  File Solid/RConn1 -- Rigid Transform8/LConn1 -- Rigid Transform9/LConn1 -- solver/RConn1 -- Rigid Transform10/LConn1 -- Rigid Transform7/LConn1 -- Transform Sensor/RConn1 -- Transform Sensor1/RConn1 -- STL frame to CoG/LConn1 -- Rigid Transform14/LConn1 -- Rigid Transform17/LConn1 -- Rigid Transform18/LConn1 -- Rigid Transform15/LConn1
  Rigid Transform15/RConn1 -- Rigid Transform5/LConn1
  UpperARM_FR/RConn1 -- Rigid Transform4/RConn1
  Rigid Transform17/RConn1 -- Rigid Transform6/LConn1
  Rigid Transform10/RConn1 -- Rigid Transform1/LConn1
  Rigid Transform18/RConn1 -- Rigid Transform11/LConn1
  Rigid Transform1/RConn1 -- LowerARM_RR/RConn1
  Rigid Transform2/LConn1 -- Rigid Transform7/RConn1
  Rigid Transform/LConn1 -- Rigid Transform8/RConn1
  Rigid Transform3/LConn1 -- Rigid Transform9/RConn1
  Rigid Transform4/LConn1 -- Rigid Transform14/RConn1
  Rigid Transform5/RConn1 -- LowerARM_FR/RConn1
  Rigid Transform6/RConn1 -- UpperARM_FL/RConn1
  Rigid Transform11/RConn1 -- LowerARM_FL/RConn1
  Simulink-PS Converter/RConn1 -- External Force and Torque/LConn1
  Simulink-PS Converter1/RConn1 -- External Force and Torque/LConn2
  Simulink-PS Converter2/RConn1 -- External Force and Torque/LConn3
  PS-Simulink Converter/LConn1 -- Transform Sensor/RConn2
  PS-Simulink Converter1/LConn1 -- Transform Sensor/RConn3
  World Frame/RConn1 -- Transform Sensor/LConn1 -- Transform Sensor1/LConn1
  STL frame to CoG/RConn1 -- External Force and Torque/RConn1
  Transform Sensor/RConn4 -- PS-Simulink Converter2/LConn1
  PS-Simulink Converter3/LConn1 -- Transform Sensor1/RConn2

== system model2bf_Chikri/Driveline ==
  Throttle (%) : Inport
  Braking (%) : Inport  Port=2
  1-D Lookup Table : Lookup_n-D  NumberOfTableDimensions=1  BreakpointsForDimension1=motor.torque_speed(:,1)  Table=motor.torque_speed(:,2)  InternalRulePriority=Speed  RndMeth=Simplest
  Acceleration calculation : Subsystem
  Demux : Demux  Outputs=3
  Gain1 : Gain  Gain=60/(2*pi)*motor.gearratio/(tyre.dynamic_radius/100)
  Scope : Scope
  Scope2 : Scope
  Subsystem2 : Subsystem
  Subsystem3 : Subsystem
  Wheel force calculation : Subsystem
  wires:
  Acceleration calculation/1(Acceleration) -> Scope2/1
  Demux/1 -> Scope/1, Gain1/1, Wheel force calculation/3(Speed (m/s)), Subsystem2/1(v (m/s))  "Speed_x"
  Subsystem3/1(MotorTrqOut (Nm)) -> Wheel force calculation/1(motor_torque)
  1-D Lookup Table/1 -> Subsystem3/1(Motor torque (Nm))
  Throttle (%)/1 -> Subsystem3/3(Throttle (%))
  Braking (%)/1 -> Subsystem2/2(Braking (%))
  Gain1/1 -> 1-D Lookup Table/1
  [Speed] -> Demux/1
  Subsystem2/1(FrictionBrake_Tr) -> Wheel force calculation/2(brake_torque)
  Subsystem2/2(RegenBrake_Tr) -> Subsystem3/2(Regen Torque)
  Wheel force calculation/1(wheel force) -> Acceleration calculation/1(wheel force)

== system model2bf_Chikri/Driver ==
  Keyboard 1 : M-S-Function  FunctionName=sfun_keyboard_input_v1_2b  mask(Keyboard Input){}
      mask help: Keyboard Input
      mask Display: fprintf('Keyboard');
  Last Key : Display
  Level-2 MATLAB S-Function : M-S-Function  FunctionName=wheelturn
  Scope1 : Scope
  aSteerWheel : Outport
  rAccelPedal : Outport  Port=2
  rBrakePedal : Outport  Port=3
  Out4 : Outport  Port=4
  wires:
  Keyboard 1/1 -> Level-2 MATLAB S-Function/1, Last Key/1, Scope1/1
  Level-2 MATLAB S-Function/1 -> aSteerWheel/1  "aSteerWheel"
  Level-2 MATLAB S-Function/3 -> rBrakePedal/1  "rBrakePedal"
  Level-2 MATLAB S-Function/2 -> rAccelPedal/1  "rAccelPedal"
  Keyboard 1/2 -> Out4/1

== system model2bf_Chikri/Driver inputs1 ==
  Throttle1 : Inport
  Brake1 : Inport  Port=2
  "\"Gas\" pedal" : simulink/Sources/Ramp  slope=0.5  start=0.5  InitialOutput=0  VectorParams1D=off
  Add : Sum  Commented=on
  Braking pedal : simulink/Sources/Ramp  Commented=on  slope=-0.4  start=0  InitialOutput=0
  Constant : Constant  Value=0
  Gain : Gain  Gain=-1
  Manual Switch : ManualSwitch
  Manual Switch1 : ManualSwitch  CurrentSetting=0
  Ramp : simulink/Sources/Ramp  Commented=on  slope=-1  start=5  InitialOutput=0
  Saturation : Saturate  UpperLimit=1  LowerLimit=0
  Saturation1 : Saturate  UpperLimit=0  LowerLimit=-1
  Saturation2 : Saturate  LowerLimit=0
  Scope : Scope
  Scope1 : Scope
  Throttle : Outport
  Braking : Outport  Port=2
  wires:
  "\"Gas\" pedal"/1 -> Saturation2/1
  Saturation2/1 -> Saturation/1
  Saturation/1 -> Manual Switch/1, Scope/1
  Manual Switch1/1 -> Braking/1
  Manual Switch/1 -> Throttle/1
  Throttle1/1 -> Manual Switch/2
  Brake1/1 -> Gain/1
  Gain/1 -> Manual Switch1/1
  Saturation1/1 -> Scope1/1, Manual Switch1/2
  Constant/1 -> Saturation1/1

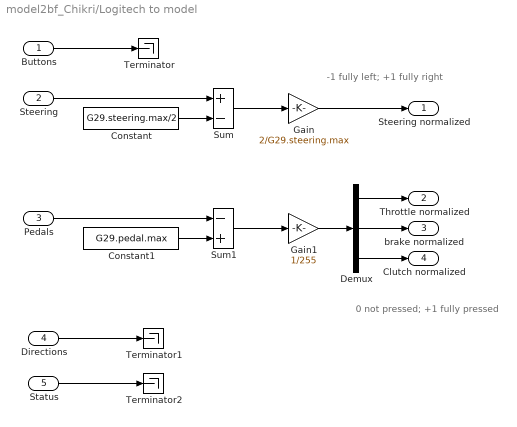
== system model2bf_Chikri/Logitech to model ==
  note: -1 fully left; +1 fully right
  note: 0 not pressed; +1 fully pressed
  Buttons : Inport
  Steering : Inport  Port=2
  Pedals : Inport  Port=3
  Directions : Inport  Port=4
  Status : Inport  Port=5
  Constant : Constant  Value=G29.steering.max/2
  Constant1 : Constant  Value=G29.pedal.max
  Demux : Demux  Outputs=3
  Gain : Gain  Gain=2/G29.steering.max
  Gain1 : Gain  Gain=1/255
  Sum : Sum  Inputs=+-
  Sum1 : Sum  Inputs=-+
  Terminator : Terminator
  Terminator1 : Terminator
  Terminator2 : Terminator
  Steering normalized : Outport
  Throttle normalized : Outport  Port=2
  brake normalized : Outport  Port=3
  Clutch normalized : Outport  Port=4
  wires:
  Buttons/1 -> Terminator/1
  Directions/1 -> Terminator1/1
  Status/1 -> Terminator2/1
  Steering/1 -> Sum/1
  Sum/1 -> Gain/1
  Constant/1 -> Sum/2
  Gain/1 -> Steering normalized/1
  Sum1/1 -> Gain1/1
  Pedals/1 -> Sum1/1
  Constant1/1 -> Sum1/2
  Gain1/1 -> Demux/1
  Demux/1 -> Throttle normalized/1
  Demux/2 -> brake normalized/1
  Demux/3 -> Clutch normalized/1
